simulink model "FOC_sim_embedded"  (R2021b)
settings: Solver=VariableStepAuto  StartTime=0.0  StopTime=SimTime  RelTol=1e-3
undefined symbols (not defined in the file): CurrCntrl_Ki, CurrCntrl_Kp, CurrCntrl_Umax, CurrCntrl_Umin, Id_ref, Iq_ref, Llr, Lls, PolePairs, RotFluxEst_Ts, RPMtoRads, Rr, Rs, Speed_ref, SVPWM_SampTs, SVPWM_SwitchTs, Tr, Ts_sim, Udc
libraries: spsIGBTDiodeLib x6, spsVoltageMeasurementLib x3, spsCurrentMeasurementLib x3, simulink x3, spsDCVoltageSourceLib x1, spsAsynchronousMachineSIUnitsLib x1, spspowerguiLib x1
settings Model: Creator=ArnóczyLászlóVince  LastModifiedBy=ArnóczyLászlóVince

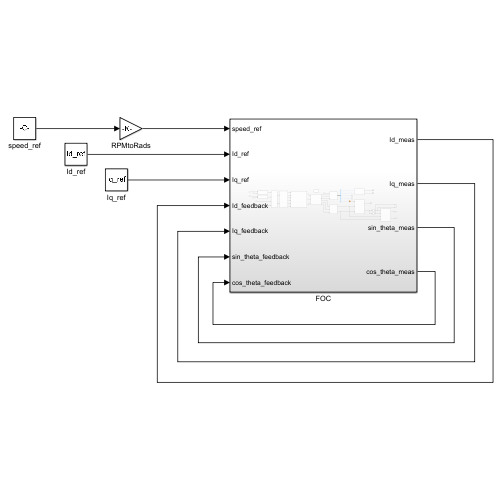
[thumbnail: Simulink's stored preview of the top-level diagram]
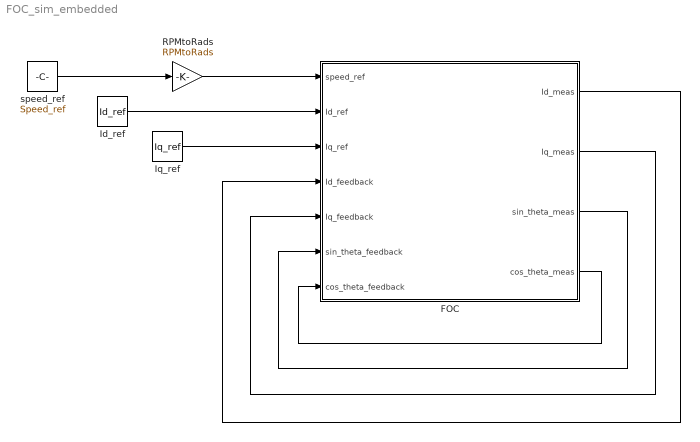
== system FOC_sim_embedded ==
  FOC : Subsystem
  Id_ref : Constant  Value=Id_ref
  Iq_ref : Constant  Value=Iq_ref
  RPMtoRads : Gain  Gain=RPMtoRads
  speed_ref : Constant  Value=Speed_ref
  wires:
  Id_ref/1 -> FOC/2(Id_ref)
  Iq_ref/1 -> FOC/3(Iq_ref)
  FOC/2(Iq_meas) -> FOC/5(Iq_feedback)
  FOC/1(Id_meas) -> FOC/4(Id_feedback)
  RPMtoRads/1 -> FOC/1(speed_ref)
  speed_ref/1 -> RPMtoRads/1
  FOC/3(sin_theta_meas) -> FOC/6(sin_theta_feedback)
  FOC/4(cos_theta_meas) -> FOC/7(cos_theta_feedback)

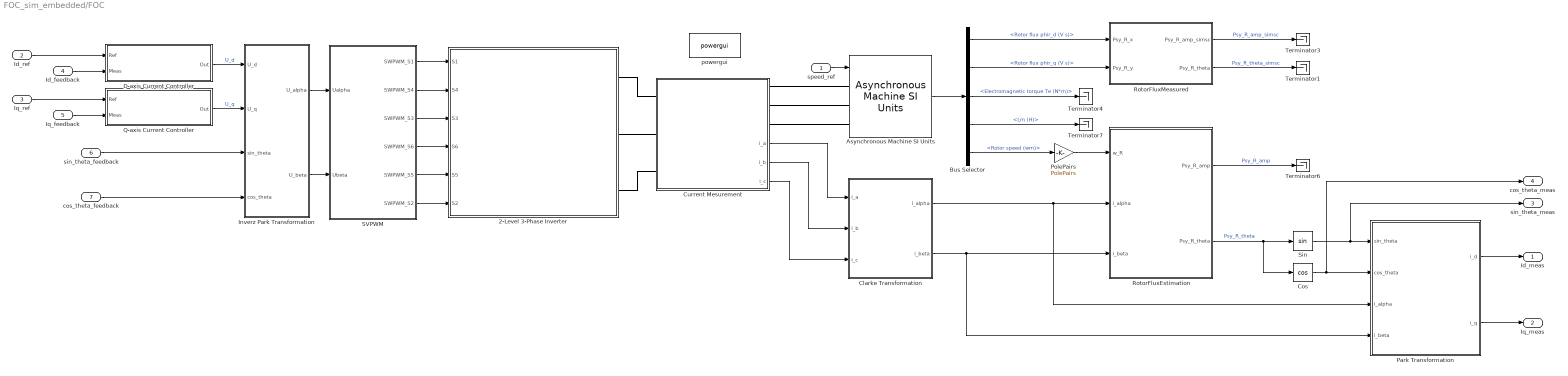
== system FOC_sim_embedded/FOC ==
  speed_ref : Inport
  Id_ref : Inport  Port=2
  Iq_ref : Inport  Port=3
  Id_feedback : Inport  Port=4
  Iq_feedback : Inport  Port=5
  sin_theta_feedback : Inport  Port=6
  cos_theta_feedback : Inport  Port=7
  2-Level 3-Phase Inverter : Subsystem
  Asynchronous Machine SI Units : spsAsynchronousMachineSIUnitsLib/Asynchronous Machine SI Units  RotorType=Squirrel-cage  PresetModel=No  MechanicalLoad=Speed w  ShowDetailedParameters=on  ReferenceFrame=Stationary  Units=SI  MeasurementBus=off  NominalParameters=[1.845e+04 400 60]  VoltageRatio=1  Stator=[Rs Lls]  Rotor=[Rr Llr]  Cage1=[0.4155 0.002066]  Cage2=[0.4168 0.0003495]  Lm=Lm  Mechanical=[0.05 0.005879 PolePairs]  PolePairs=PolePairs  InitialConditions=[0 0 0 0 0 0 0 0]  SimulateSaturation=off  Saturation=[14.03593122, 27.81365428, 53.79336849, 72.68890987, 97.98006896, 148.6815601, 215.7428561, 302.9841135, 428.7778367 ; 230, 322, 414, 460, 506, 552, 598, 644, 690]  LoadFlowParameters=1492000  TsPowergui=0  TsBlock=-1  IterativeModel=Trapezoidal non iterative  IterativeDiscreteModel=Trapezoidal non iterative  Pmec=1.492e+006
  Bus Selector : BusSelector  OutputSignals=Rotor measurements.Rotor flux phir_d (V s),Rotor measurements.Rotor flux phir_q (V s),Mechanical.Electromagnetic torque Te (N*m),Lm (H),Mechanical.Rotor speed (wm)
  Clarke Transformation : Subsystem
  Cos : Trigonometry  Operator=cos
  Current Mesurement : Subsystem
      settings: PortSchema="{\"entries\":[{\"content\":{\"sides\":[{\"content\":{\"connectorIds\":[\"LConn1\",\"LConn2\",\"LConn3\"]},\"type\":\"ConnectorPlacement.EquallySpacedRectSide\",\"uuid\":\"218ce0f1-32a4-4746-b253-7a5af0291eed\"},{\"content\":{\"connectorIds\":[\"RConn1\",\"RConn2\",\"RConn3\",\"Out1\",\"Out2\",\"Out3\"],\"side\":\"RIGHT\"},\"type\":\"ConnectorPlacement.EquallySpacedRectSide\",\"uuid\":\"ad04235a-dac5-4102-860a-7632fef99471\"},{\"content\":{\"connectorIds\":[],\"side\":\"TOP\"},\"type\":\"ConnectorPlacement.EquallySpacedRectSide\",\"uuid\":\"74b8936b-0351-412e-9dca-f97767edf200\"}]},\"type\":\"ConnectorPlacement.EquallySpacedConnector\",\"uuid\":\"d2fdc9e1-fb80-48b0-9a83-205876194764\"}],\"packageUris\":[\"http://schema.mathworks.com/mf0/Connector/R2020b\"],\"version\":\"1.0\"}"
  D-axis Current Controller : Subsystem
  Inverz Park Transformation : Subsystem
  Park Transformation : Subsystem
  PolePairs : Gain  Gain=PolePairs
  Q-axis Current Controller : Subsystem
  RotorFluxEstimation : Subsystem
  RotorFluxMeasured : Subsystem
  SVPWM : Subsystem
  Sin : Trigonometry
  Terminator{1,3..4,6..7} (5 alike) : Terminator
  powergui : spspowerguiLib/powergui  Priority=1  SimulationMode=Discrete  SampleTime=Ts_sim  frequency=60  Iterations=50  frequencyindice=0  Pbase=100e6  ErrMax=1e-4  UnitsV=kV  UnitsW=MW  buscounter=0  FunctionMessages=off  echomessages=off  EnableUseOfTLC=off  CurrentSourceSwitches=off  DisableSnubberDevices=off  DisableRonSwitches=off  DisableVfSwitches=off  DisplayEquations=off  AutomaticDiscreteSolvers=off  SolverType=Tustin/Backward Euler (TBE)  Interpol=off  ExternalGateDelay=off  methode=off  Ts=100  x0status=blocks  SPID=on  SwTol=0  HookPort=off  NonlinearTolerance=1e-4  nMaxIteration=100  ContinueOnMaxIteration=off  RestoreLinks=warning  ResistiveCurrentMeasurement=off  Frange=[0:2:500]  Ylog=off  Xlog=on  ShowGrid=off  save=off  variable=ZData  structure=0  ZoomFFT=off  StartTime=0.0  cycles=1  DisplayStyle=1  fundamental=60  FreqAxis=off  MaxFrequency=1000  frequencyindicesteady=1  RmsSteady=1  display=off
  Id_meas : Outport
  Iq_meas : Outport  Port=2
  sin_theta_meas : Outport  Port=3
  cos_theta_meas : Outport  Port=4
  wires:
  Inverz Park Transformation/1(U_alpha) -> SVPWM/1(Ualpha)
  cos_theta_feedback/1 -> Inverz Park Transformation/4(cos_theta)
  D-axis Current Controller/1(Out) -> Inverz Park Transformation/1(U_d)  "U_d"
  Id_ref/1 -> D-axis Current Controller/1(Ref)
  PolePairs/1 -> RotorFluxEstimation/1(w_R)
  Bus Selector/2 -> RotorFluxMeasured/2(Psy_R_y)  "<Rotor flux phir_q (V s)>"
  Bus Selector/3 -> Terminator4/1  "<Electromagnetic torque Te (N*m)>"
  Iq_ref/1 -> Q-axis Current Controller/1(Ref)
  SVPWM/4(SWPWM_S6) -> 2-Level 3-Phase Inverter/4(S6)
  RotorFluxEstimation/1(Psy_R_amp) -> Terminator6/1  "Psy_R_amp"
  RotorFluxMeasured/2(Psy_R_theta) -> Terminator1/1  "Psy_R_theta_simsc"
  RotorFluxMeasured/1(Psy_R_amp_simsc) -> Terminator3/1  "Psy_R_amp_simsc"
  Q-axis Current Controller/1(Out) -> Inverz Park Transformation/2(U_q)  "U_q"
  Bus Selector/1 -> RotorFluxMeasured/1(Psy_R_x)  "<Rotor flux phir_d (V s)>"
  SVPWM/6(SWPWM_S2) -> 2-Level 3-Phase Inverter/6(S2)
  SVPWM/3(SWPWM_S3) -> 2-Level 3-Phase Inverter/3(S3)
  SVPWM/1(SWPWM_S1) -> 2-Level 3-Phase Inverter/1(S1)
  speed_ref/1 -> Asynchronous Machine SI Units/1
  Clarke Transformation/1(i_alpha) -> Park Transformation/3(i_alpha), RotorFluxEstimation/2(i_alpha)
  Clarke Transformation/2(i_beta) -> Park Transformation/4(i_beta), RotorFluxEstimation/3(i_beta)
  Inverz Park Transformation/2(U_beta) -> SVPWM/2(Ubeta)
  Asynchronous Machine SI Units/1 -> Bus Selector/1
  SVPWM/2(SWPWM_S4) -> 2-Level 3-Phase Inverter/2(S4)
  SVPWM/5(SWPWM_S5) -> 2-Level 3-Phase Inverter/5(S5)
  Bus Selector/5 -> PolePairs/1  "<Rotor speed (wm)>"
  sin_theta_feedback/1 -> Inverz Park Transformation/3(sin_theta)
  Park Transformation/1(i_d) -> Id_meas/1
  Park Transformation/2(i_q) -> Iq_meas/1
  Iq_feedback/1 -> Q-axis Current Controller/2(Meas)
  Id_feedback/1 -> D-axis Current Controller/2(Meas)
  RotorFluxEstimation/2(Psy_R_theta) -> Cos/1, Sin/1  "Psy_R_theta"
  Sin/1 -> sin_theta_meas/1, Park Transformation/1(sin_theta)
  Cos/1 -> cos_theta_meas/1, Park Transformation/2(cos_theta)
  Bus Selector/4 -> Terminator7/1  "<Lm (H)>"
  Current Mesurement/1(i_a) -> Clarke Transformation/1(i_a)
  Current Mesurement/2(i_b) -> Clarke Transformation/2(i_b)
  Current Mesurement/3(i_c) -> Clarke Transformation/3(i_c)
  connections:
  Current Mesurement/LConn1 -- 2-Level 3-Phase Inverter/RConn1
  Current Mesurement/LConn2 -- 2-Level 3-Phase Inverter/RConn2
  Current Mesurement/LConn3 -- 2-Level 3-Phase Inverter/RConn3
  Current Mesurement/RConn2 -- Asynchronous Machine SI Units/LConn2
  Current Mesurement/RConn1 -- Asynchronous Machine SI Units/LConn1
  Current Mesurement/RConn3 -- Asynchronous Machine SI Units/LConn3

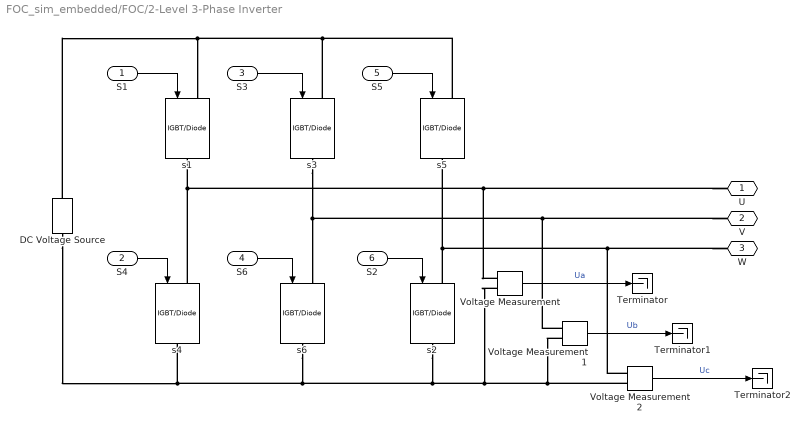
== system FOC_sim_embedded/FOC/2-Level 3-Phase Inverter ==
  S1 : Inport
  S4 : Inport  Port=2
  S3 : Inport  Port=3
  S6 : Inport  Port=4
  S5 : Inport  Port=5
  S2 : Inport  Port=6
  DC Voltage Source : spsDCVoltageSourceLib/DC Voltage Source  Amplitude=Udc  Measurements=None
  Terminator : Terminator
  Terminator1 : Terminator
  Terminator2 : Terminator
  Voltage Measurement : spsVoltageMeasurementLib/Voltage Measurement  PhasorSimulation=off  OutputType=Complex  PSBequivalent=0
  Voltage Measurement1 : spsVoltageMeasurementLib/Voltage Measurement  PhasorSimulation=off  OutputType=Complex  PSBequivalent=0
  Voltage Measurement2 : spsVoltageMeasurementLib/Voltage Measurement  PhasorSimulation=off  OutputType=Complex  PSBequivalent=0
  s{1..6} (6 alike) : spsIGBTDiodeLib/IGBT//Diode  Ron=1e-3  Rs=1e5  Cs=inf  Measurements=off
  U : PMIOPort  Side=Right
  V : PMIOPort  Port=2  Side=Right
  W : PMIOPort  Port=3  Side=Right
  wires:
  Voltage Measurement1/1 -> Terminator1/1  "Ub"
  S6/1 -> s6/1
  S1/1 -> s1/1
  Voltage Measurement2/1 -> Terminator2/1  "Uc"
  S4/1 -> s4/1
  S2/1 -> s2/1
  Voltage Measurement/1 -> Terminator/1  "Ua"
  S5/1 -> s5/1
  S3/1 -> s3/1
  connections:
  s5/RConn1 -- s2/LConn1 -- W/RConn1 -- Voltage Measurement2/LConn1
  Voltage Measurement1/LConn1 -- V/RConn1 -- s3/RConn1 -- s6/LConn1
  Voltage Measurement1/LConn2 -- Voltage Measurement/LConn2 -- s2/RConn1 -- s6/RConn1 -- DC Voltage Source/LConn1 -- s4/RConn1 -- Voltage Measurement2/LConn2
  s1/RConn1 -- s4/LConn1 -- U/RConn1 -- Voltage Measurement/LConn1
  s5/LConn1 -- s3/LConn1 -- DC Voltage Source/RConn1 -- s1/LConn1

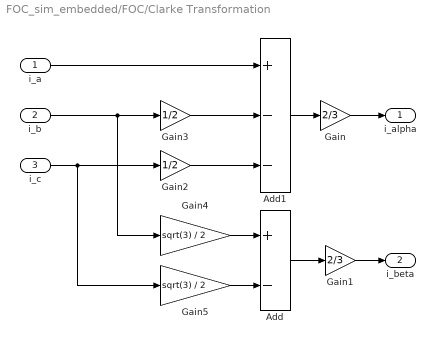
== system FOC_sim_embedded/FOC/Clarke Transformation ==
  i_a : Inport
  i_b : Inport  Port=2
  i_c : Inport  Port=3
  Add : Sum  Inputs=+-
  Add1 : Sum  Inputs=+--
  Gain : Gain  Gain=2/3
  Gain1 : Gain  Gain=2/3
  Gain2 : Gain  Gain=1/2
  Gain3 : Gain  Gain=1/2
  Gain4 : Gain  Gain=sqrt(3) / 2
  Gain5 : Gain  Gain=sqrt(3) / 2
  i_alpha : Outport
  i_beta : Outport  Port=2
  wires:
  Gain4/1 -> Add/1
  Add/1 -> Gain1/1
  i_a/1 -> Add1/1
  Gain5/1 -> Add/2
  Add1/1 -> Gain/1
  Gain2/1 -> Add1/3
  Gain3/1 -> Add1/2
  i_b/1 -> Gain4/1, Gain3/1
  i_c/1 -> Gain5/1, Gain2/1
  Gain1/1 -> i_beta/1
  Gain/1 -> i_alpha/1

== system FOC_sim_embedded/FOC/Current Mesurement ==
  Current Measurement : spsCurrentMeasurementLib/Current Measurement  PhasorSimulation=off  OutputType=Complex  PSBequivalent=0
  Current Measurement1 : spsCurrentMeasurementLib/Current Measurement  PhasorSimulation=off  OutputType=Complex  PSBequivalent=0
  Current Measurement2 : spsCurrentMeasurementLib/Current Measurement  PhasorSimulation=off  OutputType=Complex  PSBequivalent=0
  U : PMIOPort  Side=Left
  V : PMIOPort  Port=2  Side=Left
  W : PMIOPort  Port=3  Side=Left
  U_mot : PMIOPort  Port=4  Side=Right
  V_mot : PMIOPort  Port=5  Side=Right
  W_mot : PMIOPort  Port=6  Side=Right
  i_a : Outport
  i_b : Outport  Port=2
  i_c : Outport  Port=3
  wires:
  Current Measurement1/1 -> i_b/1  "I_b"
  Current Measurement/1 -> i_a/1  "I_a"
  Current Measurement2/1 -> i_c/1  "I_c"
  connections:
  Current Measurement/LConn1 -- U/RConn1
  V_mot/RConn1 -- Current Measurement1/RConn1
  Current Measurement1/LConn1 -- V/RConn1
  W_mot/RConn1 -- Current Measurement2/RConn1
  U_mot/RConn1 -- Current Measurement/RConn1
  Current Measurement2/LConn1 -- W/RConn1

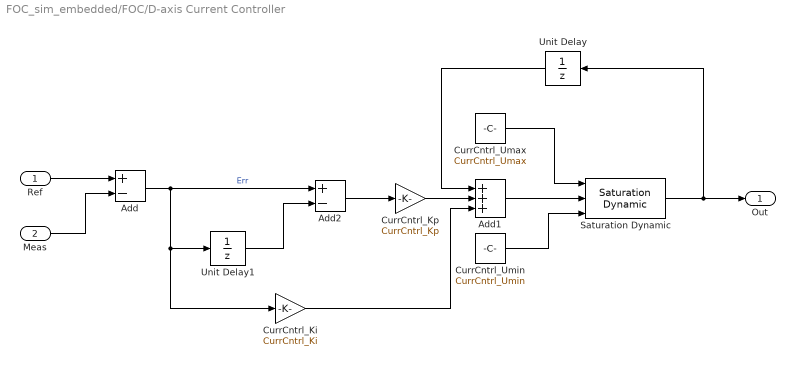
== system FOC_sim_embedded/FOC/D-axis Current Controller ==
  Ref : Inport
  Meas : Inport  Port=2
  Add : Sum  Inputs=+-
  Add1 : Sum  Inputs=+++
  Add2 : Sum  Inputs=+-
  CurrCntrl_Ki : Gain  Gain=CurrCntrl_Ki
  CurrCntrl_Kp : Gain  Gain=CurrCntrl_Kp
  CurrCntrl_Umax : Constant  Value=CurrCntrl_Umax
  CurrCntrl_Umin : Constant  Value=CurrCntrl_Umin
  Saturation Dynamic : simulink/Discontinuities/Saturation Dynamic  OutMin=[]  OutMax=[]  OutDataTypeStr=Inherit: Same as second input  OutDataType=fixdt(1, 16)  OutScaling=2^-10  DoSatur=off
  Unit Delay : UnitDelay  SampleTime=-1  HasFrameUpgradeWarning=on
  Unit Delay1 : UnitDelay  SampleTime=-1  HasFrameUpgradeWarning=on
  Out : Outport
  wires:
  CurrCntrl_Ki/1 -> Add1/3
  Ref/1 -> Add/1
  Meas/1 -> Add/2
  Add/1 -> Add2/1, Unit Delay1/1, CurrCntrl_Ki/1  "Err"
  Unit Delay1/1 -> Add2/2
  Add2/1 -> CurrCntrl_Kp/1
  CurrCntrl_Kp/1 -> Add1/2
  Add1/1 -> Saturation Dynamic/2
  CurrCntrl_Umax/1 -> Saturation Dynamic/1
  CurrCntrl_Umin/1 -> Saturation Dynamic/3
  Saturation Dynamic/1 -> Unit Delay/1, Out/1
  Unit Delay/1 -> Add1/1

== system FOC_sim_embedded/FOC/Inverz Park Transformation ==
  U_d : Inport
  U_q : Inport  Port=2
  sin_theta : Inport  Port=3
  cos_theta : Inport  Port=4
  Add1 : Sum  Inputs=+-
  Add2 : Sum
  Product{,1..3} (4 alike) : Product
  U_alpha : Outport
  U_beta : Outport  Port=2
  wires:
  Product/1 -> Add1/1
  Product2/1 -> Add2/2
  U_d/1 -> Product3/2, Product/2
  Product1/1 -> Add1/2
  Product3/1 -> Add2/1
  U_q/1 -> Product2/1, Product1/1
  Add2/1 -> U_beta/1
  Add1/1 -> U_alpha/1
  cos_theta/1 -> Product2/2, Product/1
  sin_theta/1 -> Product3/1, Product1/2

== system FOC_sim_embedded/FOC/Park Transformation ==
  sin_theta : Inport
  cos_theta : Inport  Port=2
  i_alpha : Inport  Port=3
  i_beta : Inport  Port=4
  Add1 : Sum
  Add2 : Sum  Inputs=-+
  Product{,1..3} (4 alike) : Product
  i_d : Outport
  i_q : Outport  Port=2
  wires:
  Product/1 -> Add1/1
  Add1/1 -> i_d/1
  Product1/1 -> Add1/2
  cos_theta/1 -> Product2/2, Product/1
  Add2/1 -> i_q/1
  i_alpha/1 -> Product/2, Product3/2
  Product3/1 -> Add2/1
  Product2/1 -> Add2/2
  sin_theta/1 -> Product3/1, Product1/2
  i_beta/1 -> Product2/1, Product1/1

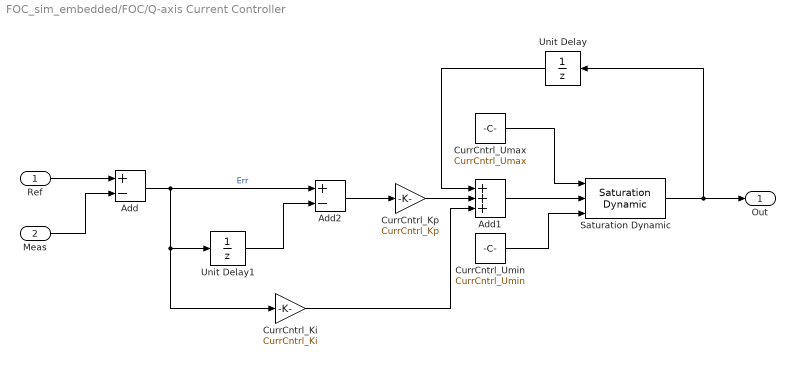
== system FOC_sim_embedded/FOC/Q-axis Current Controller ==
  Ref : Inport
  Meas : Inport  Port=2
  Add : Sum  Inputs=+-
  Add1 : Sum  Inputs=+++
  Add2 : Sum  Inputs=+-
  CurrCntrl_Ki : Gain  Gain=CurrCntrl_Ki
  CurrCntrl_Kp : Gain  Gain=CurrCntrl_Kp
  CurrCntrl_Umax : Constant  Value=CurrCntrl_Umax
  CurrCntrl_Umin : Constant  Value=CurrCntrl_Umin
  Saturation Dynamic : simulink/Discontinuities/Saturation Dynamic  OutMin=[]  OutMax=[]  OutDataTypeStr=Inherit: Same as second input  OutDataType=fixdt(1, 16)  OutScaling=2^-10  DoSatur=off
  Unit Delay : UnitDelay  SampleTime=-1  HasFrameUpgradeWarning=on
  Unit Delay1 : UnitDelay  SampleTime=-1  HasFrameUpgradeWarning=on
  Out : Outport
  wires:
  CurrCntrl_Ki/1 -> Add1/3
  Ref/1 -> Add/1
  Meas/1 -> Add/2
  Add/1 -> Add2/1, Unit Delay1/1, CurrCntrl_Ki/1  "Err"
  Unit Delay1/1 -> Add2/2
  Add2/1 -> CurrCntrl_Kp/1
  CurrCntrl_Kp/1 -> Add1/2
  Add1/1 -> Saturation Dynamic/2
  CurrCntrl_Umax/1 -> Saturation Dynamic/1
  CurrCntrl_Umin/1 -> Saturation Dynamic/3
  Saturation Dynamic/1 -> Unit Delay/1, Out/1
  Unit Delay/1 -> Add1/1

== system FOC_sim_embedded/FOC/RotorFluxEstimation ==
  w_R : Inport
  i_alpha : Inport  Port=2
  i_beta : Inport  Port=3
  PsyR_Amp_Calc : Subsystem
  PsyR_Amp_angle : Subsystem
  PsyR_XY_calc : Subsystem
  Psy_R_amp : Outport
  Psy_R_theta : Outport  Port=2
  wires:
  w_R/1 -> PsyR_XY_calc/2(w_R)
  i_beta/1 -> PsyR_XY_calc/3(i_S_ y)
  i_alpha/1 -> PsyR_XY_calc/1(i_S_ x)
  PsyR_Amp_Calc/1(Psy_R_amp) -> Psy_R_amp/1
  PsyR_Amp_angle/1(Psy_R_theta) -> Psy_R_theta/1
  PsyR_XY_calc/1(Psy_R_ x) -> PsyR_Amp_angle/1(Psy_R_ x), PsyR_Amp_Calc/1(Psy_R_ x)
  PsyR_XY_calc/2(Psy_R_ y) -> PsyR_Amp_Calc/2(Psy_R_ y), PsyR_Amp_angle/2(Psy_R_ y)

== system FOC_sim_embedded/FOC/RotorFluxMeasured ==
  Psy_R_x : Inport
  Psy_R_y : Inport  Port=2
  PsyR_Amp_Calc : Subsystem
  PsyR_Amp_angle : Subsystem
  Psy_R_amp_simsc : Outport
  Psy_R_theta : Outport  Port=2
  wires:
  PsyR_Amp_angle/1(Psy_R_theta) -> Psy_R_theta/1
  PsyR_Amp_Calc/1(Psy_R_amp_simsc) -> Psy_R_amp_simsc/1
  Psy_R_x/1 -> PsyR_Amp_Calc/1(Psy_x), PsyR_Amp_angle/1(Psy_R_ x)
  Psy_R_y/1 -> PsyR_Amp_Calc/2(Psy_y), PsyR_Amp_angle/2(Psy_R_ y)

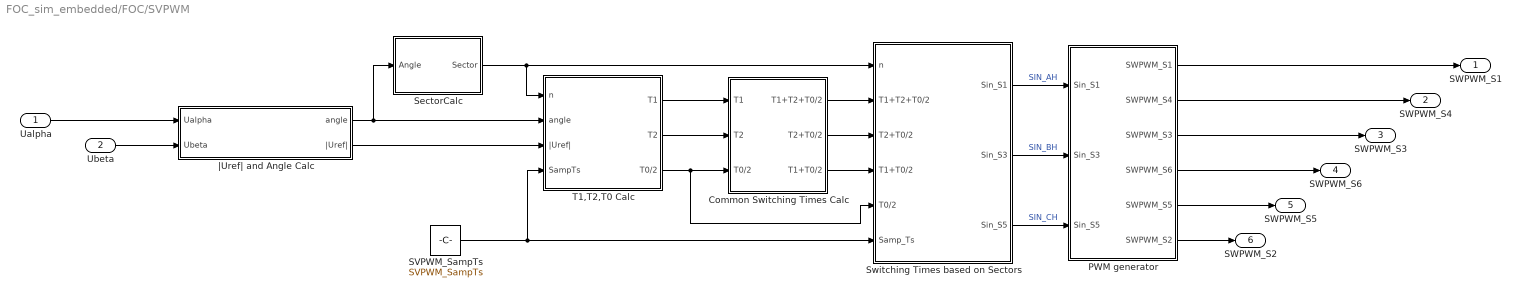
== system FOC_sim_embedded/FOC/SVPWM ==
  Ualpha : Inport
  Ubeta : Inport  Port=2
  " SectorCalc" : Subsystem
  Common Switching Times Calc : Subsystem
  PWM generator : Subsystem
  SVPWM_SampTs : Constant  Value=SVPWM_SampTs
  "Switching Times based on Sectors " : Subsystem
  T1,T2,T0 Calc : Subsystem
  |Uref| and Angle Calc : Subsystem
  SWPWM_S1 : Outport
  SWPWM_S4 : Outport  Port=2
  SWPWM_S3 : Outport  Port=3
  SWPWM_S6 : Outport  Port=4
  SWPWM_S5 : Outport  Port=5
  SWPWM_S2 : Outport  Port=6
  wires:
  " SectorCalc"/1(Sector) -> T1,T2,T0 Calc/1(n), "Switching Times based on Sectors "/1(n)
  SVPWM_SampTs/1 -> T1,T2,T0 Calc/4(SampTs), "Switching Times based on Sectors "/6(Samp_Ts)
  "Switching Times based on Sectors "/3(Sin_S5) -> PWM generator/3(Sin_S5)  "SIN_CH"
  PWM generator/2(SWPWM_S4) -> SWPWM_S4/1
  T1,T2,T0 Calc/1(T1) -> Common Switching Times Calc/1(T1)
  "Switching Times based on Sectors "/2(Sin_S3) -> PWM generator/2(Sin_S3)  "SIN_BH"
  Common Switching Times Calc/2(T2+T0/2) -> "Switching Times based on Sectors "/3(T2+T0/2)
  Common Switching Times Calc/3(T1+T0/2) -> "Switching Times based on Sectors "/4(T1+T0/2)
  |Uref| and Angle Calc/1(angle) -> T1,T2,T0 Calc/2(angle), " SectorCalc"/1(Angle)
  |Uref| and Angle Calc/2(|Uref|) -> T1,T2,T0 Calc/3(|Uref|)
  "Switching Times based on Sectors "/1(Sin_S1) -> PWM generator/1(Sin_S1)  "SIN_AH"
  T1,T2,T0 Calc/2(T2) -> Common Switching Times Calc/2(T2)
  Common Switching Times Calc/1(T1+T2+T0/2) -> "Switching Times based on Sectors "/2(T1+T2+T0/2)
  PWM generator/3(SWPWM_S3) -> SWPWM_S3/1
  PWM generator/4(SWPWM_S6) -> SWPWM_S6/1
  PWM generator/6(SWPWM_S2) -> SWPWM_S2/1
  PWM generator/5(SWPWM_S5) -> SWPWM_S5/1
  PWM generator/1(SWPWM_S1) -> SWPWM_S1/1
  T1,T2,T0 Calc/3(T0/2) -> "Switching Times based on Sectors "/5(T0/2), Common Switching Times Calc/3(T0/2)
  Ubeta/1 -> |Uref| and Angle Calc/2(Ubeta)
  Ualpha/1 -> |Uref| and Angle Calc/1(Ualpha)

== system FOC_sim_embedded/FOC/RotorFluxEstimation/PsyR_Amp_Calc ==
  Psy_R_ x : Inport
  Psy_R_ y : Inport  Port=2
  Add2 : Sum
  Sqrt : Sqrt  SaturateOnIntegerOverflow=on
  Square : Math  Operator=square  SaturateOnIntegerOverflow=on
  Square1 : Math  Operator=square  SaturateOnIntegerOverflow=on
  Psy_R_amp : Outport
  wires:
  Psy_R_ y/1 -> Square/1
  Square/1 -> Add2/1
  Psy_R_ x/1 -> Square1/1
  Square1/1 -> Add2/2
  Add2/1 -> Sqrt/1
  Sqrt/1 -> Psy_R_amp/1

== system FOC_sim_embedded/FOC/RotorFluxEstimation/PsyR_Amp_angle ==
  Psy_R_ x : Inport
  Psy_R_ y : Inport  Port=2
  Tan : Trigonometry  Operator=atan2
  Psy_R_theta : Outport
  wires:
  Psy_R_ y/1 -> Tan/1
  Tan/1 -> Psy_R_theta/1
  Psy_R_ x/1 -> Tan/2

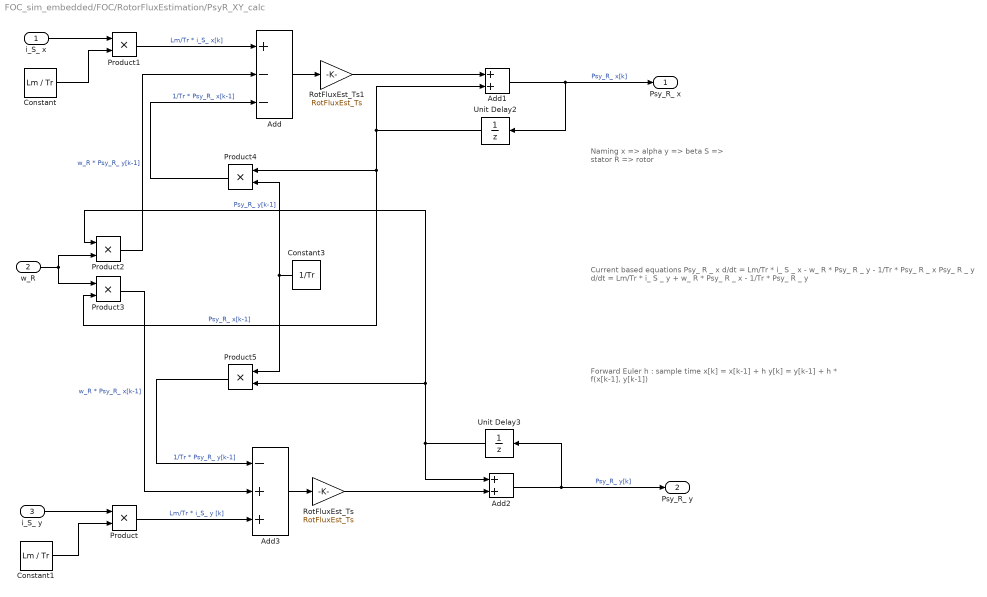
== system FOC_sim_embedded/FOC/RotorFluxEstimation/PsyR_XY_calc ==
  note: Forward Euler
      | h : sample time
      | x[k] = x[k-1] + h
      | y[k] = y[k-1] + h * f(x[k-1], y[k-1])
  note: Current based equations
      | Psy_ R _ x d/dt = Lm/Tr * i_ S _ x - w_ R * Psy_ R _ y - 1/Tr * Psy_ R _ x
      | Psy_ R _ y d/dt = Lm/Tr * i_ S _ y + w_ R * Psy_ R _ x - 1/Tr * Psy_ R _ y
  note: Naming
      |
      | x => alpha
      | y => beta
      | S => stator
      | R => rotor
  i_S_ x : Inport
  w_R : Inport  Port=2
  i_S_ y : Inport  Port=3
  Add : Sum  Inputs=+--
  Add1 : Sum
  Add2 : Sum
  Add3 : Sum  Inputs=-++
  Constant : Constant  Value=Lm / Tr
  Constant1 : Constant  Value=Lm / Tr
  Constant3 : Constant  Value=1/Tr
  Product{,1..5} (6 alike) : Product
  RotFluxEst_Ts : Gain  Gain=RotFluxEst_Ts
  RotFluxEst_Ts1 : Gain  Gain=RotFluxEst_Ts
  Unit Delay2 : UnitDelay  SampleTime=-1  HasFrameUpgradeWarning=on
  Unit Delay3 : UnitDelay  SampleTime=-1  HasFrameUpgradeWarning=on
  Psy_R_ x : Outport
  Psy_R_ y : Outport  Port=2
  wires:
  Unit Delay2/1 -> Product4/1, Product3/2, Add1/2  "Psy_R_ x[k-1]"
  Add3/1 -> RotFluxEst_Ts/1
  w_R/1 -> Product3/1, Product2/2
  Constant1/1 -> Product/2
  i_S_ y/1 -> Product/1
  Product2/1 -> Add/2  "w_R * Psy_R_ y[k-1]"
  Add/1 -> RotFluxEst_Ts1/1
  Product1/1 -> Add/1  "Lm/Tr * i_S_ x[k]"
  Product4/1 -> Add/3  "1/Tr * Psy_R_ x[k-1]"
  Constant3/1 -> Product5/1, Product4/2
  Product5/1 -> Add3/1  "1/Tr * Psy_R_ y[k-1]"
  Product3/1 -> Add3/2  "w_R * Psy_R_ x[k-1]"
  Product/1 -> Add3/3  "Lm/Tr * i_S_ y [k]"
  i_S_ x/1 -> Product1/1
  Constant/1 -> Product1/2
  Add1/1 -> Psy_R_ x/1, Unit Delay2/1  "Psy_R_ x[k]"
  Add2/1 -> Psy_R_ y/1, Unit Delay3/1  "Psy_R_ y[k]"
  Unit Delay3/1 -> Product5/2, Product2/1, Add2/1  "Psy_R_ y[k-1]"
  RotFluxEst_Ts/1 -> Add2/2
  RotFluxEst_Ts1/1 -> Add1/1

== system FOC_sim_embedded/FOC/RotorFluxMeasured/PsyR_Amp_Calc ==
  Psy_x : Inport
  Psy_y : Inport  Port=2
  Add2 : Sum
  Sqrt : Sqrt  SaturateOnIntegerOverflow=on
  Square : Math  Operator=square  SaturateOnIntegerOverflow=on
  Square1 : Math  Operator=square  SaturateOnIntegerOverflow=on
  Psy_R_amp_simsc : Outport
  wires:
  Add2/1 -> Sqrt/1
  Square/1 -> Add2/1
  Square1/1 -> Add2/2
  Psy_y/1 -> Square1/1
  Sqrt/1 -> Psy_R_amp_simsc/1
  Psy_x/1 -> Square/1

== system FOC_sim_embedded/FOC/RotorFluxMeasured/PsyR_Amp_angle ==
  Psy_R_ x : Inport
  Psy_R_ y : Inport  Port=2
  Tan : Trigonometry  Operator=atan2
  Psy_R_theta : Outport
  wires:
  Psy_R_ y/1 -> Tan/1
  Tan/1 -> Psy_R_theta/1
  Psy_R_ x/1 -> Tan/2

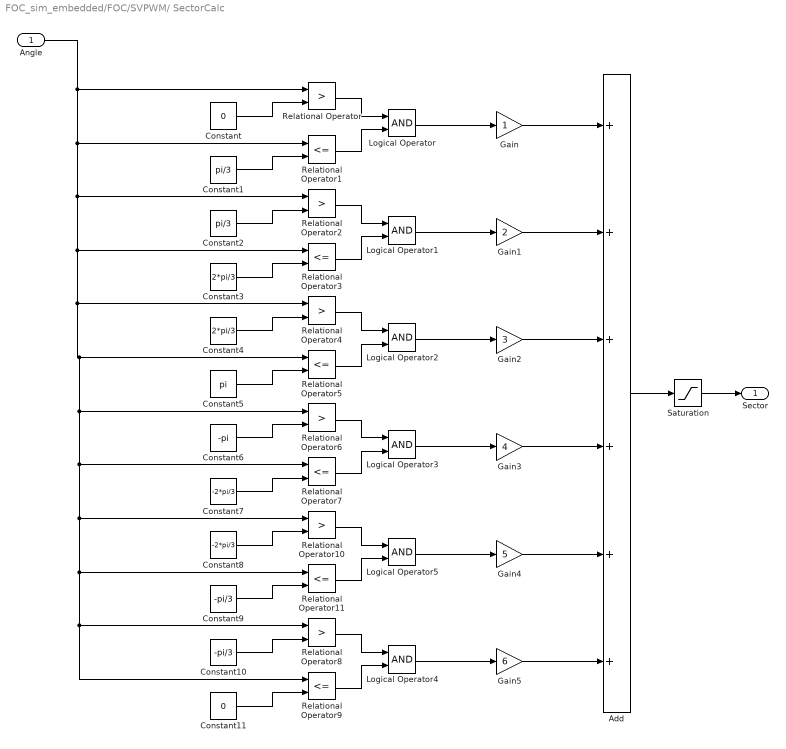
== system FOC_sim_embedded/FOC/SVPWM/ SectorCalc ==
  Angle : Inport
  Add : Sum  Inputs=++++++
  Constant : Constant  Value=0
  Constant1 : Constant  Value=pi/3
  Constant10 : Constant  Value=-pi/3
  Constant11 : Constant  Value=0
  Constant2 : Constant  Value=pi/3
  Constant3 : Constant  Value=2*pi/3
  Constant4 : Constant  Value=2*pi/3
  Constant5 : Constant  Value=pi
  Constant6 : Constant  Value=-pi
  Constant7 : Constant  Value=-2*pi/3
  Constant8 : Constant  Value=-2*pi/3
  Constant9 : Constant  Value=-pi/3
  Gain : Gain
  Gain1 : Gain  Gain=2
  Gain2 : Gain  Gain=3
  Gain3 : Gain  Gain=4
  Gain4 : Gain  Gain=5
  Gain5 : Gain  Gain=6
  Logical Operator{,1..5} (6 alike) : Logic  AllPortsSameDT=off  OutDataTypeStr=boolean
  Relational Operator{,2,4,6,8,10} (6 alike) : RelationalOperator  Operator=>  OutDataTypeStr=boolean  RndMeth=Simplest
  Relational Operator{1,3,5,7,9,11} (6 alike) : RelationalOperator  Operator=<=  OutDataTypeStr=boolean  RndMeth=Simplest
  Saturation : Saturate  UpperLimit=6  LowerLimit=1
  Sector : Outport
  wires:
  Relational Operator/1 -> Logical Operator/1
  Relational Operator1/1 -> Logical Operator/2
  Angle/1 -> Relational Operator9/1, Relational Operator8/1, Relational Operator11/1, Relational Operator10/1, Relational Operator7/1, Relational Operator6/1, Relational Operator5/1, Relational Operator4/1, Relational Operator3/1, Relational Operator2/1, Relational Operator1/1, Relational Operator/1
  Relational Operator2/1 -> Logical Operator1/1
  Relational Operator3/1 -> Logical Operator1/2
  Relational Operator4/1 -> Logical Operator2/1
  Relational Operator5/1 -> Logical Operator2/2
  Relational Operator6/1 -> Logical Operator3/1
  Relational Operator7/1 -> Logical Operator3/2
  Relational Operator8/1 -> Logical Operator4/1
  Relational Operator9/1 -> Logical Operator4/2
  Relational Operator10/1 -> Logical Operator5/1
  Relational Operator11/1 -> Logical Operator5/2
  Logical Operator/1 -> Gain/1
  Logical Operator1/1 -> Gain1/1
  Logical Operator2/1 -> Gain2/1
  Logical Operator3/1 -> Gain3/1
  Logical Operator5/1 -> Gain4/1
  Logical Operator4/1 -> Gain5/1
  Gain/1 -> Add/1
  Gain1/1 -> Add/2
  Gain2/1 -> Add/3
  Gain3/1 -> Add/4
  Gain4/1 -> Add/5
  Gain5/1 -> Add/6
  Constant/1 -> Relational Operator/2
  Constant1/1 -> Relational Operator1/2
  Constant2/1 -> Relational Operator2/2
  Constant3/1 -> Relational Operator3/2
  Constant4/1 -> Relational Operator4/2
  Constant5/1 -> Relational Operator5/2
  Constant6/1 -> Relational Operator6/2
  Constant7/1 -> Relational Operator7/2
  Constant8/1 -> Relational Operator10/2
  Constant9/1 -> Relational Operator11/2
  Constant10/1 -> Relational Operator8/2
  Constant11/1 -> Relational Operator9/2
  Add/1 -> Saturation/1
  Saturation/1 -> Sector/1

== system FOC_sim_embedded/FOC/SVPWM/Common Switching Times Calc ==
  T1 : Inport
  T2 : Inport  Port=2
  T0/2 : Inport  Port=3
  Add : Sum
  Add1 : Sum
  Add3 : Sum
  T1+T2+T0/2 : Outport
  T2+T0/2 : Outport  Port=2
  T1+T0/2 : Outport  Port=3
  wires:
  Add/1 -> T2+T0/2/1, Add3/2
  Add1/1 -> T1+T0/2/1
  Add3/1 -> T1+T2+T0/2/1
  T1/1 -> Add3/1, Add1/1
  T2/1 -> Add/2
  T0/2/1 -> Add/1, Add1/2

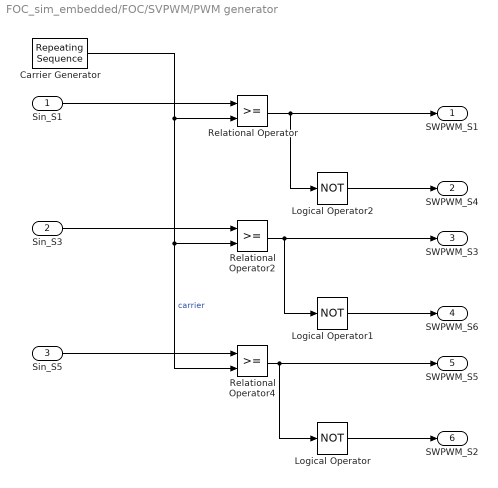
== system FOC_sim_embedded/FOC/SVPWM/PWM generator ==
  Sin_S1 : Inport
  Sin_S3 : Inport  Port=2
  Sin_S5 : Inport  Port=3
  Carrier Generator : simulink/Sources/Repeating Sequence  rep_seq_t="[0  SVPWM_SwitchTs/2 SVPWM_SwitchTs ]"  rep_seq_y="[  0 1 0 ]"
  Logical Operator : Logic  Operator=NOT  AllPortsSameDT=off  OutDataTypeStr=boolean
  Logical Operator1 : Logic  Operator=NOT  AllPortsSameDT=off  OutDataTypeStr=boolean
  Logical Operator2 : Logic  Operator=NOT  AllPortsSameDT=off  OutDataTypeStr=boolean
  Relational Operator : RelationalOperator  OutDataTypeStr=boolean  RndMeth=Simplest
  Relational Operator2 : RelationalOperator  OutDataTypeStr=boolean  RndMeth=Simplest
  Relational Operator4 : RelationalOperator  OutDataTypeStr=boolean  RndMeth=Simplest
  SWPWM_S1 : Outport
  SWPWM_S4 : Outport  Port=2
  SWPWM_S3 : Outport  Port=3
  SWPWM_S6 : Outport  Port=4
  SWPWM_S5 : Outport  Port=5
  SWPWM_S2 : Outport  Port=6
  wires:
  Sin_S1/1 -> Relational Operator/1
  Sin_S3/1 -> Relational Operator2/1
  Sin_S5/1 -> Relational Operator4/1
  Relational Operator/1 -> Logical Operator2/1, SWPWM_S1/1
  Relational Operator2/1 -> SWPWM_S3/1, Logical Operator1/1
  Relational Operator4/1 -> SWPWM_S5/1, Logical Operator/1
  Logical Operator1/1 -> SWPWM_S6/1
  Logical Operator2/1 -> SWPWM_S4/1
  Logical Operator/1 -> SWPWM_S2/1
  Carrier Generator/1 -> Relational Operator4/2, Relational Operator2/2, Relational Operator/2  "carrier"

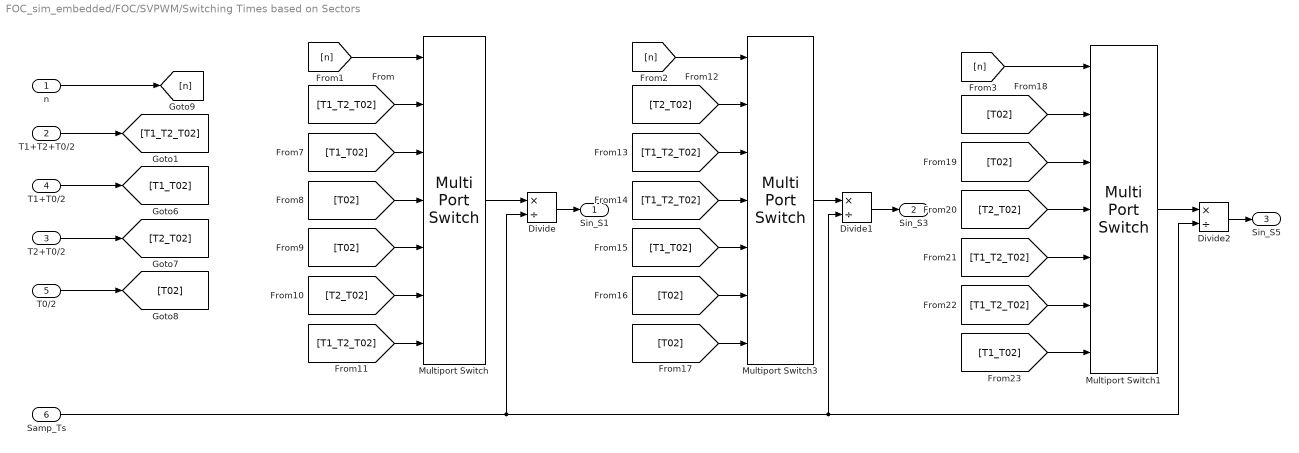
== system FOC_sim_embedded/FOC/SVPWM/Switching Times based on Sectors  ==
  n : Inport
  T1+T2+T0/2 : Inport  Port=2
  T2+T0/2 : Inport  Port=3
  T1+T0/2 : Inport  Port=4
  T0/2 : Inport  Port=5
  Samp_Ts : Inport  Port=6
  Divide : Product  Inputs=*/
  Divide1 : Product  Inputs=*/
  Divide2 : Product  Inputs=*/
  Multiport Switch : MultiPortSwitch  DataPortOrder=Specify indices  Inputs=6  DataPortIndices={1,2,3,4,5,6}  DiagnosticForDefault=None
  Multiport Switch1 : MultiPortSwitch  DataPortOrder=Specify indices  Inputs=6  DataPortIndices={1,2,3,4,5,6}  DiagnosticForDefault=None
  Multiport Switch3 : MultiPortSwitch  DataPortOrder=Specify indices  Inputs=6  DataPortIndices={1,2,3,4,5,6}  DiagnosticForDefault=None
  Sin_S1 : Outport
  Sin_S3 : Outport  Port=2
  Sin_S5 : Outport  Port=3
  wires:
  [n] -> Multiport Switch/1
  [n] -> Multiport Switch3/1
  [T1_T2_T02] -> Multiport Switch/7
  [T1_T2_T02] -> Multiport Switch3/3
  [T02] -> Multiport Switch/4
  [T02] -> Multiport Switch/5
  [T1_T2_T02] -> Multiport Switch/2
  [T1_T2_T02] -> Multiport Switch3/4
  [T02] -> Multiport Switch3/7
  [T1_T02] -> Multiport Switch1/7
  [T2_T02] -> Multiport Switch1/4
  [T02] -> Multiport Switch1/3
  [T1_T02] -> Multiport Switch3/5
  [T1_T2_T02] -> Multiport Switch1/5
  [T2_T02] -> Multiport Switch3/2
  [T02] -> Multiport Switch1/2
  [T1_T02] -> Multiport Switch/3
  [T2_T02] -> Multiport Switch/6
  [T02] -> Multiport Switch3/6
  [T1_T2_T02] -> Multiport Switch1/6
  [n] -> Multiport Switch1/1
  n/1 -> [n]
  T1+T2+T0/2/1 -> [T1_T2_T02]
  T1+T0/2/1 -> [T1_T02]
  T2+T0/2/1 -> [T2_T02]
  T0/2/1 -> [T02]
  Samp_Ts/1 -> Divide/2, Divide2/2, Divide1/2
  Divide/1 -> Sin_S1/1
  Multiport Switch/1 -> Divide/1
  Multiport Switch3/1 -> Divide1/1
  Divide1/1 -> Sin_S3/1
  Divide2/1 -> Sin_S5/1
  Multiport Switch1/1 -> Divide2/1

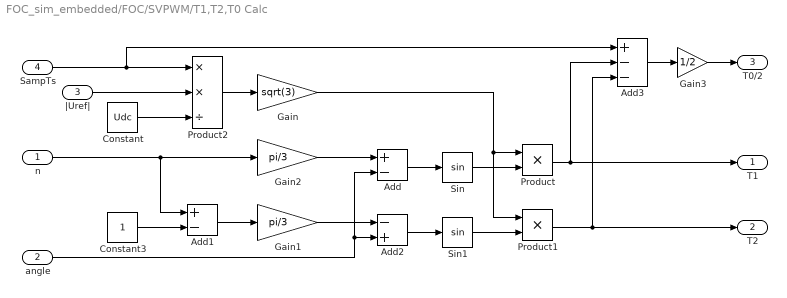
== system FOC_sim_embedded/FOC/SVPWM/T1,T2,T0 Calc ==
  n : Inport
  angle : Inport  Port=2
  |Uref| : Inport  Port=3
  SampTs : Inport  Port=4
  Add : Sum  Inputs=+-
  Add1 : Sum  Inputs=+-
  Add2 : Sum  Inputs=-+
  Add3 : Sum  Inputs=+--
  Constant : Constant  Value=Udc
  Constant3 : Constant
  Gain : Gain  Gain=sqrt(3)
  Gain1 : Gain  Gain=pi/3
  Gain2 : Gain  Gain=pi/3
  Gain3 : Gain  Gain=1/2
  Product : Product
  Product1 : Product
  Product2 : Product  Inputs=**/
  Sin : Trigonometry
  Sin1 : Trigonometry
  T1 : Outport
  T2 : Outport  Port=2
  T0/2 : Outport  Port=3
  wires:
  |Uref|/1 -> Product2/2
  Gain2/1 -> Add/1
  Add/1 -> Sin/1
  Product2/1 -> Gain/1
  Sin/1 -> Product/2
  Product/1 -> T1/1, Add3/2
  Sin1/1 -> Product1/2
  n/1 -> Gain2/1, Add1/1
  Add1/1 -> Gain1/1
  Constant3/1 -> Add1/2
  Add2/1 -> Sin1/1
  Product1/1 -> T2/1, Add3/3
  Add3/1 -> Gain3/1
  SampTs/1 -> Add3/1, Product2/1
  Gain/1 -> Product/1, Product1/1
  angle/1 -> Add/2, Add2/2
  Gain1/1 -> Add2/1
  Gain3/1 -> T0/2/1
  Constant/1 -> Product2/3

== system FOC_sim_embedded/FOC/SVPWM/|Uref| and Angle Calc ==
  Ualpha : Inport
  Ubeta : Inport  Port=2
  Add : Sum
  Sqrt : Sqrt  SaturateOnIntegerOverflow=on
  Square : Math  Operator=square  OutputSignalType=real  SaturateOnIntegerOverflow=on
  Square1 : Math  Operator=square  OutputSignalType=real  SaturateOnIntegerOverflow=on
  Trigonometric Function : Trigonometry  Operator=atan2
  angle : Outport
  |Uref| : Outport  Port=2
  wires:
  Sqrt/1 -> |Uref|/1  "vref"
  Trigonometric Function/1 -> angle/1  "angle"
  Ualpha/1 -> Square/1, Trigonometric Function/2
  Ubeta/1 -> Trigonometric Function/1, Square1/1
  Square/1 -> Add/1
  Square1/1 -> Add/2
  Add/1 -> Sqrt/1
